simulink model "sim_initseq_example"  (Simulink 8.1)
settings: Solver=FixedStepDiscrete  StartTime=0.0  StopTime=5.0  FixedStep=1  RelTol=1e-3
libraries: simulink x4
settings Model: Creator=gcampa  LastModifiedBy=gcampa
settings OptimizationCC: ExpressionDepthLimit=128
settings DebuggingCC: FcnCallInpInsideContextMsg=EnableAllAsWarning

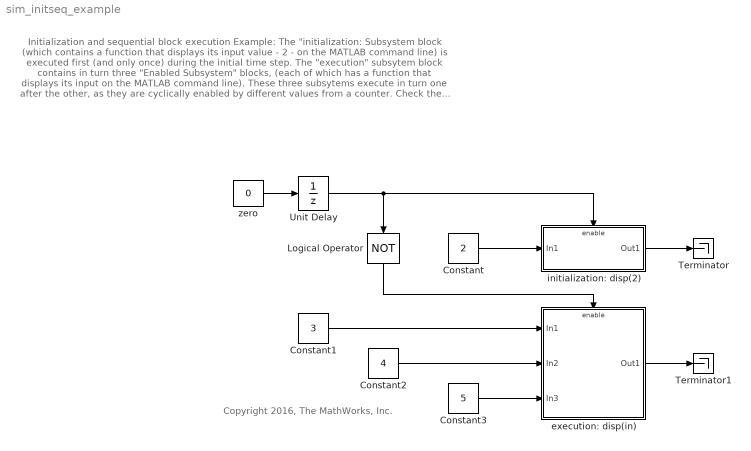
== system sim_initseq_example ==
  note: Initialization and sequential block execution Example:
      |
      | The "initialization: Subsystem block (which contains a function that displays its input value - 2 - on the
      | MATLAB command line) is executed first (and only once) during the initial time step.
      |
      | The "execution" subsytem block contains in turn three "Enabled Subsystem" blocks, (each of which
      | has a function that displays its input on the MATLAB command line). These three subsytems execute
      | in turn one after the other, as they are cyclically enabled by different values from a counter.
      |
      | Check the MATLAB command line to confirm the proper execution order.
  note: Copyright 2016, The MathWorks, Inc.
  Constant : Constant  Value=2
  Constant1 : Constant  Value=3
  Constant2 : Constant  Value=4
  Constant3 : Constant  Value=5
  Logical Operator : Logic  Operator=NOT  AllPortsSameDT=off  OutDataTypeStr=boolean
  Terminator : Terminator
  Terminator1 : Terminator
  Unit Delay : UnitDelay  InitialCondition=1  SampleTime=-1
  execution: disp(in) : Subsystem  TreatAsAtomicUnit=on
  initialization: disp(2) : Subsystem  TreatAsAtomicUnit=on
  zero : Constant  Value=0
  wires:
  zero/1 -> Unit Delay/1
  Unit Delay/1 -> Logical Operator/1, initialization: disp(2)/Enable
  Constant/1 -> initialization: disp(2)/1(In1)
  Logical Operator/1 -> execution: disp(in)/Enable
  Constant1/1 -> execution: disp(in)/1(In1)
  initialization: disp(2)/1(Out1) -> Terminator/1
  execution: disp(in)/1(Out1) -> Terminator1/1
  Constant2/1 -> execution: disp(in)/2(In2)
  Constant3/1 -> execution: disp(in)/3(In3)

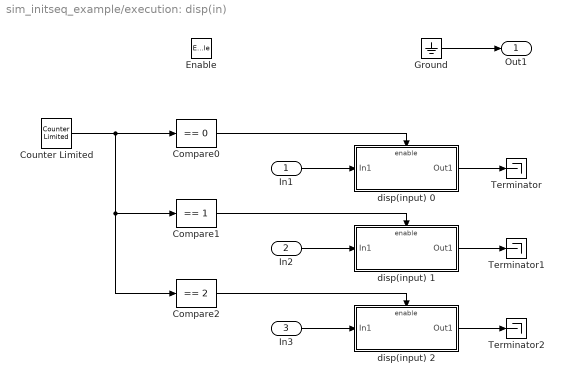
== system sim_initseq_example/execution: disp(in) ==
  In1 : Inport
  In2 : Inport  Port=2
  In3 : Inport  Port=3
  Enable : EnablePort
  Compare0 : simulink/Logic and Bit Operations/Compare To Constant  relop===  const=0  LogicOutDataTypeMode=uint8
  Compare1 : simulink/Logic and Bit Operations/Compare To Constant  relop===  const=1  LogicOutDataTypeMode=uint8
  Compare2 : simulink/Logic and Bit Operations/Compare To Constant  relop===  const=2  LogicOutDataTypeMode=uint8
  Counter Limited : simulink/Sources/Counter Limited  uplimit=2  tsamp=-1
  Ground : Ground
  Terminator : Terminator
  Terminator1 : Terminator
  Terminator2 : Terminator
  disp(input) 0 : Subsystem  TreatAsAtomicUnit=on
  disp(input) 1 : Subsystem  TreatAsAtomicUnit=on
  disp(input) 2 : Subsystem  TreatAsAtomicUnit=on
  Out1 : Outport
  wires:
  In1/1 -> disp(input) 0/1(In1)
  Ground/1 -> Out1/1
  In2/1 -> disp(input) 1/1(In1)
  disp(input) 0/1(Out1) -> Terminator/1
  disp(input) 1/1(Out1) -> Terminator1/1
  In3/1 -> disp(input) 2/1(In1)
  disp(input) 2/1(Out1) -> Terminator2/1
  Counter Limited/1 -> Compare2/1, Compare1/1, Compare0/1
  Compare0/1 -> disp(input) 0/Enable
  Compare1/1 -> disp(input) 1/Enable
  Compare2/1 -> disp(input) 2/Enable

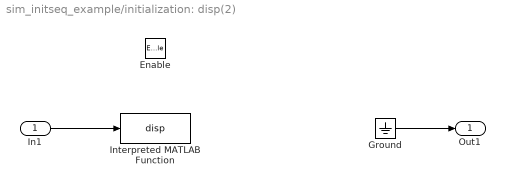
== system sim_initseq_example/initialization: disp(2) ==
  In1 : Inport
  Enable : EnablePort
  Ground : Ground
  Interpreted MATLAB Function : MATLABFcn  MATLABFcn=disp  OutputDimensions=0
  Out1 : Outport
  wires:
  Ground/1 -> Out1/1
  In1/1 -> Interpreted MATLAB Function/1

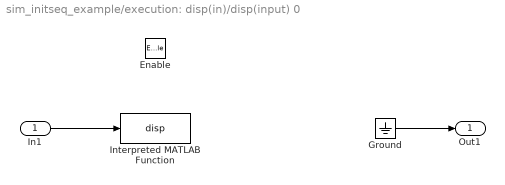
== system sim_initseq_example/execution: disp(in)/disp(input) 0 ==
  In1 : Inport
  Enable : EnablePort
  Ground : Ground
  Interpreted MATLAB Function : MATLABFcn  MATLABFcn=disp  OutputDimensions=0
  Out1 : Outport
  wires:
  In1/1 -> Interpreted MATLAB Function/1
  Ground/1 -> Out1/1

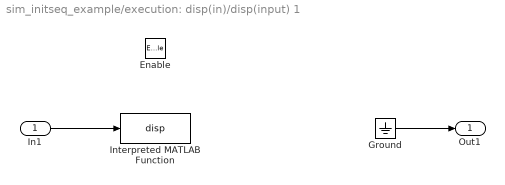
== system sim_initseq_example/execution: disp(in)/disp(input) 1 ==
  In1 : Inport
  Enable : EnablePort
  Ground : Ground
  Interpreted MATLAB Function : MATLABFcn  MATLABFcn=disp  OutputDimensions=0
  Out1 : Outport
  wires:
  Ground/1 -> Out1/1
  In1/1 -> Interpreted MATLAB Function/1

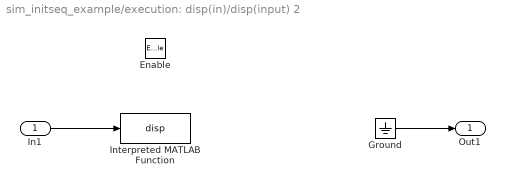
== system sim_initseq_example/execution: disp(in)/disp(input) 2 ==
  In1 : Inport
  Enable : EnablePort
  Ground : Ground
  Interpreted MATLAB Function : MATLABFcn  MATLABFcn=disp  OutputDimensions=0
  Out1 : Outport
  wires:
  In1/1 -> Interpreted MATLAB Function/1
  Ground/1 -> Out1/1
